simulink model "sum_collapse_bool_test"  (Simulink 8.7)
settings: Solver=VariableStepDiscrete  StartTime=0.0  StopTime=10.0  RelTol=1e-3
settings Model: Creator=arnaud  LastModifiedBy=hamza
settings DataIOCC: SaveFormat=Structure  SignalLoggingSaveFormat=ModelDataLogs
settings OptimizationCC: ExpressionDepthLimit=2147483647
settings DebuggingCC: SolverPrmCheckMsg=warning  FcnCallInpInsideContextMsg=UseLocalSettings  StateNameClashWarn=warning  StrictBusMsg=Warning
settings GRTTargetCC: GeneratePreprocessorConditionals=Use local settings  CombineOutputUpdateFcns=off  GRTInterface=on

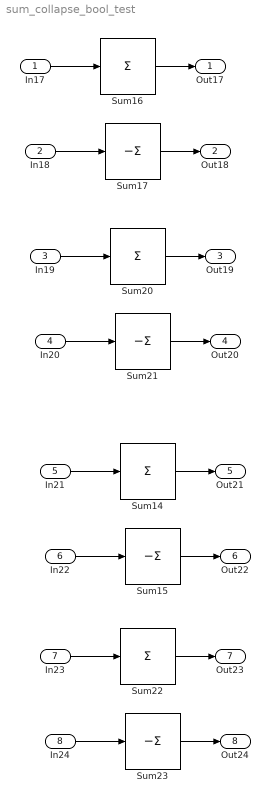
== system sum_collapse_bool_test ==
  In17 : Inport  OutDataTypeStr=int32
  In18 : Inport  Port=2  OutDataTypeStr=int32
  In19 : Inport  Port=3  OutDataTypeStr=int32  PortDimensions=3
  In20 : Inport  Port=4  OutDataTypeStr=int32  PortDimensions=3
  In21 : Inport  Port=5  OutDataTypeStr=int32  PortDimensions=[2 3]
  In22 : Inport  Port=6  OutDataTypeStr=int32  PortDimensions=[2 3]
  In23 : Inport  Port=7  OutDataTypeStr=int32  PortDimensions=[2 3]
  In24 : Inport  Port=8  OutDataTypeStr=int32  PortDimensions=[2 3]
  Sum14 : Sum  Inputs=+  CollapseMode=Specified dimension
  Sum15 : Sum  Inputs=-  CollapseMode=Specified dimension
  Sum16 : Sum  Inputs=+  CollapseMode=Specified dimension
  Sum17 : Sum  Inputs=-  CollapseMode=Specified dimension
  Sum20 : Sum  Inputs=+  CollapseMode=Specified dimension
  Sum21 : Sum  Inputs=-  CollapseMode=Specified dimension
  Sum22 : Sum  Inputs=+  CollapseMode=Specified dimension  CollapseDim=2
  Sum23 : Sum  Inputs=-  CollapseMode=Specified dimension  CollapseDim=2
  Out17 : Outport
  Out18 : Outport  Port=2
  Out19 : Outport  Port=3
  Out20 : Outport  Port=4
  Out21 : Outport  Port=5
  Out22 : Outport  Port=6
  Out23 : Outport  Port=7
  Out24 : Outport  Port=8
  wires:
  In17/1 -> Sum16/1
  Sum16/1 -> Out17/1
  In18/1 -> Sum17/1
  Sum17/1 -> Out18/1
  In19/1 -> Sum20/1
  Sum20/1 -> Out19/1
  In20/1 -> Sum21/1
  Sum21/1 -> Out20/1
  In21/1 -> Sum14/1
  Sum14/1 -> Out21/1
  In22/1 -> Sum15/1
  Sum15/1 -> Out22/1
  In23/1 -> Sum22/1
  Sum22/1 -> Out23/1
  In24/1 -> Sum23/1
  Sum23/1 -> Out24/1
